simulink model "fullcontroller"  (R2024a)
settings: Solver=VariableStepAuto  StartTime=0.0  StopTime=5  RelTol=1e-3
undefined symbols (not defined in the file): al, al2, D, detect_delay, gear, J, K_b, K_t, Kp, kptr, kptr2, L, M, R, taud, taud2, taui, tautr, tautr2, Ts, wb, Wrad, wzi
settings Model: Creator=Emil  LastModifiedBy=Emil

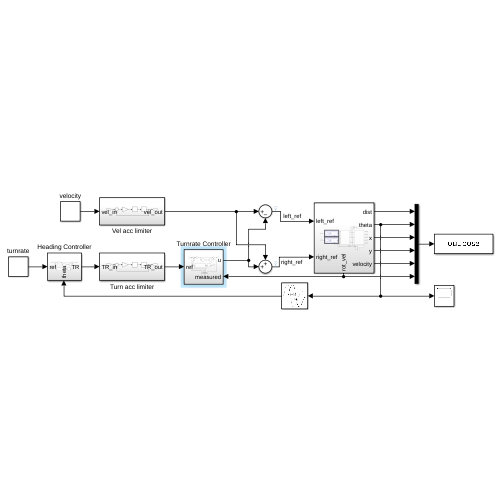
[thumbnail: Simulink's stored preview of the top-level diagram]
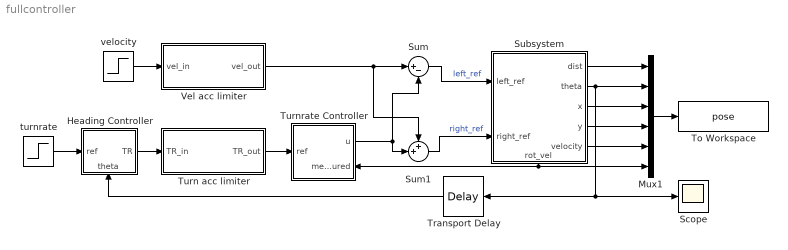
== system fullcontroller ==
  Heading Controller : Subsystem
      settings: PortSchema="{\"entries\":[{\"content\":{\"sides\":[{\"content\":{\"connectorIds\":[\"In1\"]},\"type\":\"ConnectorPlacement.EquallySpacedRectSide\",\"uuid\":\"b11ff20e-e335-4cf4-8322-1741fc0eb0d9\"},{\"content\":{\"connectorIds\":[\"Out1\"],\"side\":\"RIGHT\"},\"type\":\"ConnectorPlacement.EquallySpacedRectSide\",\"uuid\":\"fac384a7-55d1-4174-bfba-2626770ec520\"},{\"content\":{\"side\":\"TOP\"},\"type\":\"ConnectorPlacement.EquallySpacedRectSide\",\"uuid\":\"e325242d-1aa0-49ab-831d-5f009ebdd3a1\"},{\"content\":{\"connectorIds\":[\"In2\"],\"side\":\"BOTTOM\"},\"type\":\"ConnectorPlacement.EquallySpacedRectSide\",\"uuid\":\"ecba5a56-1e6f-49a1-b044-0798465cfff3\"}]},\"type\":\"ConnectorPlacement.EquallySpacedConnector\",\"uuid\":\"e06c607b-bc81-4732-8f37-206b6429b87f\"}],\"packageUris\":[\"http://schema.mathworks.com/mf0/Connector/R2020b\"],\"version\":\"1.0\"}"
  Mux1 : Mux  Inputs=6
  Scope : Scope
  Subsystem : Subsystem
      settings: PortSchema="{\"entries\":[{\"content\":{\"sides\":[{\"content\":{\"connectorIds\":[\"In1\",\"In2\"]},\"type\":\"ConnectorPlacement.EquallySpacedRectSide\",\"uuid\":\"e07b1068-606a-48e5-99f8-ac206fedc370\"},{\"content\":{\"connectorIds\":[\"Out1\",\"Out2\",\"Out3\",\"Out4\",\"Out5\"],\"side\":\"RIGHT\"},\"type\":\"ConnectorPlacement.EquallySpacedRectSide\",\"uuid\":\"74f7c964-e43c-4a5c-b857-64620296c31d\"},{\"content\":{\"side\":\"TOP\"},\"type\":\"ConnectorPlacement.EquallySpacedRectSide\",\"uuid\":\"331776cf-0fe9-40bc-a7d3-a5362462a3b4\"},{\"content\":{\"connectorIds\":[\"Out6\"],\"side\":\"BOTTOM\"},\"type\":\"ConnectorPlacement.EquallySpacedRectSide\",\"uuid\":\"defae528-7c87-433c-80d2-64239180a36e\"}]},\"type\":\"ConnectorPlacement.EquallySpacedConnector\",\"uuid\":\"4a46fe46-5a27-417e-b483-15ad12e25037\"}],\"packageUris\":[\"http://schema.mathworks.com/mf0/Connector/R2020b\"],\"version\":\"1.0\"}"
  Sum : Sum  Inputs=|+-
  Sum1 : Sum  Inputs=++|
  To Workspace : ToWorkspace  VariableName=pose  SaveFormat=Timeseries  SampleTime=-1
  Transport Delay : TransportDelay  DelayTime=detect_delay
  Turn acc limiter : Subsystem
  Turnrate Controller : Subsystem
      settings: PortSchema="{\"entries\":[{\"content\":{\"sides\":[{\"content\":{\"connectorIds\":[\"In1\"]},\"type\":\"ConnectorPlacement.EquallySpacedRectSide\",\"uuid\":\"51bc9059-e822-41b0-ad9a-58a8b0ba50e6\"},{\"content\":{\"connectorIds\":[\"Out1\",\"In2\"],\"side\":\"RIGHT\"},\"type\":\"ConnectorPlacement.EquallySpacedRectSide\",\"uuid\":\"f66c1df7-72f8-4460-aff3-9c1b28d487c9\"},{\"content\":{\"side\":\"TOP\"},\"type\":\"ConnectorPlacement.EquallySpacedRectSide\",\"uuid\":\"4a1b057f-a482-47d5-80e1-886b48e9d90a\"},{\"content\":{\"side\":\"BOTTOM\"},\"type\":\"ConnectorPlacement.EquallySpacedRectSide\",\"uuid\":\"a3ca5889-e809-4546-84f7-a1327d7aedb2\"}]},\"type\":\"ConnectorPlacement.EquallySpacedConnector\",\"uuid\":\"471e63b8-cc27-4ade-a003-f77fbe7d347a\"}],\"packageUris\":[\"http://schema.mathworks.com/mf0/Connector/R2020b\"],\"version\":\"1.0\"}"
  Vel acc limiter : Subsystem
  turnrate : Step  After=0.1  SampleTime=0
  velocity : Step  Time=0.05  After=0.1  SampleTime=0
  wires:
  Mux1/1 -> To Workspace/1
  Turn acc limiter/1(TR_out) -> Turnrate Controller/1(ref)
  velocity/1 -> Vel acc limiter/1(vel_in)
  Vel acc limiter/1(vel_out) -> Sum1/1, Sum/1
  Turnrate Controller/1(u) -> Sum1/2, Sum/2
  Sum/1 -> Subsystem/1(left_ref)  "left_ref"
  Sum1/1 -> Subsystem/2(right_ref)  "right_ref"
  Subsystem/1(dist) -> Mux1/1
  Subsystem/2(theta) -> Scope/1, Transport Delay/1, Mux1/2
  Subsystem/3(x) -> Mux1/3
  Subsystem/6(rot_vel) -> Turnrate Controller/2(measured), Mux1/6
  Subsystem/4(y) -> Mux1/4
  Subsystem/5(velocity) -> Mux1/5
  Heading Controller/1(TR) -> Turn acc limiter/1(TR_in)
  turnrate/1 -> Heading Controller/1(ref)
  Transport Delay/1 -> Heading Controller/2(theta)

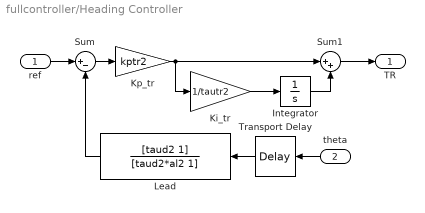
== system fullcontroller/Heading Controller ==
  ref : Inport
  theta : Inport  Port=2
  Integrator : Integrator
  Ki_tr : Gain  Gain=1/tautr2
  Kp_tr : Gain  Gain=kptr2
  Lead : TransferFcn  Numerator=[taud2 1]  Denominator=[taud2*al2 1]
  Sum : Sum  Inputs=|+-
  Sum1 : Sum  Inputs=|++
  Transport Delay : TransportDelay  DelayTime=detect_delay
  TR : Outport
  wires:
  theta/1 -> Transport Delay/1
  Transport Delay/1 -> Lead/1
  Lead/1 -> Sum/2
  Sum/1 -> Kp_tr/1
  Kp_tr/1 -> Sum1/1, Ki_tr/1
  Sum1/1 -> TR/1
  Ki_tr/1 -> Integrator/1
  Integrator/1 -> Sum1/2
  ref/1 -> Sum/1

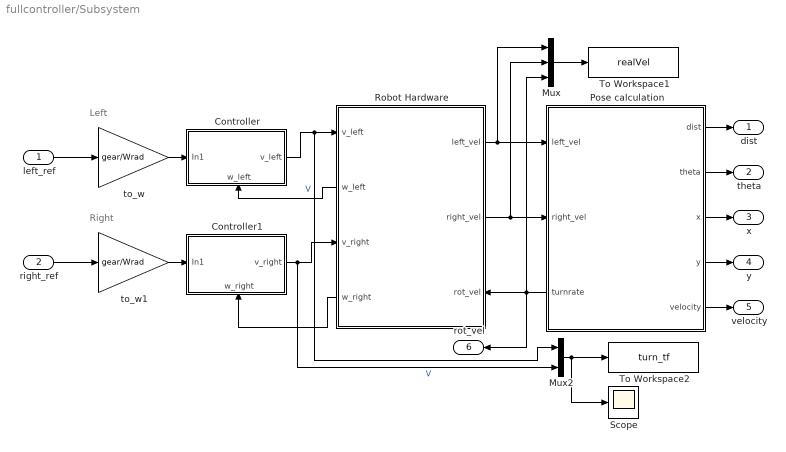
== system fullcontroller/Subsystem ==
  note: Left
  note: Right
  left_ref : Inport
  right_ref : Inport  Port=2
  Controller : Subsystem
      settings: PortSchema="{\"entries\":[{\"content\":{\"sides\":[{\"content\":{\"connectorIds\":[\"In1\"]},\"type\":\"ConnectorPlacement.EquallySpacedRectSide\",\"uuid\":\"2261268e-b6d1-4642-b5b2-9c0d266891c3\"},{\"content\":{\"connectorIds\":[\"Out1\"],\"side\":\"RIGHT\"},\"type\":\"ConnectorPlacement.EquallySpacedRectSide\",\"uuid\":\"4cfe3340-c893-4897-944b-2b0f290aa09a\"},{\"content\":{\"side\":\"TOP\"},\"type\":\"ConnectorPlacement.EquallySpacedRectSide\",\"uuid\":\"7108c253-9182-4668-b671-097ac861718f\"},{\"content\":{\"connectorIds\":[\"In2\"],\"side\":\"BOTTOM\"},\"type\":\"ConnectorPlacement.EquallySpacedRectSide\",\"uuid\":\"922d98a4-0301-4faa-ad82-d40d0b91da64\"}]},\"type\":\"ConnectorPlacement.EquallySpacedConnector\",\"uuid\":\"919d27b6-1b02-4194-927e-2efe9a2a427e\"}],\"packageUris\":[\"http://schema.mathworks.com/mf0/Connector/R2020b\"],\"version\":\"1.0\"}"
  Controller1 : Subsystem
      settings: PortSchema="{\"entries\":[{\"content\":{\"sides\":[{\"content\":{\"connectorIds\":[\"In1\"]},\"type\":\"ConnectorPlacement.EquallySpacedRectSide\",\"uuid\":\"2261268e-b6d1-4642-b5b2-9c0d266891c3\"},{\"content\":{\"connectorIds\":[\"Out1\"],\"side\":\"RIGHT\"},\"type\":\"ConnectorPlacement.EquallySpacedRectSide\",\"uuid\":\"4cfe3340-c893-4897-944b-2b0f290aa09a\"},{\"content\":{\"side\":\"TOP\"},\"type\":\"ConnectorPlacement.EquallySpacedRectSide\",\"uuid\":\"7108c253-9182-4668-b671-097ac861718f\"},{\"content\":{\"connectorIds\":[\"In2\"],\"side\":\"BOTTOM\"},\"type\":\"ConnectorPlacement.EquallySpacedRectSide\",\"uuid\":\"922d98a4-0301-4faa-ad82-d40d0b91da64\"}]},\"type\":\"ConnectorPlacement.EquallySpacedConnector\",\"uuid\":\"919d27b6-1b02-4194-927e-2efe9a2a427e\"}],\"packageUris\":[\"http://schema.mathworks.com/mf0/Connector/R2020b\"],\"version\":\"1.0\"}"
  Mux : Mux  Inputs=3
  Mux2 : Mux  Inputs=2
  Pose calculation : Subsystem
      settings: PortSchema="{\"entries\":[{\"content\":{\"sides\":[{\"content\":{\"connectorIds\":[\"In1\",\"In2\",\"Out6\"]},\"type\":\"ConnectorPlacement.EquallySpacedRectSide\",\"uuid\":\"bee664ca-7f8c-44aa-b52f-15284e139093\"},{\"content\":{\"connectorIds\":[\"Out1\",\"Out2\",\"Out3\",\"Out4\",\"Out5\"],\"side\":\"RIGHT\"},\"type\":\"ConnectorPlacement.EquallySpacedRectSide\",\"uuid\":\"08237290-c5a4-4af9-9089-e794091ff74a\"},{\"content\":{\"side\":\"TOP\"},\"type\":\"ConnectorPlacement.EquallySpacedRectSide\",\"uuid\":\"b1c152cf-47fe-475d-84d8-7839de8b0ea3\"}]},\"type\":\"ConnectorPlacement.EquallySpacedConnector\",\"uuid\":\"8442b5c9-5ac9-43e4-9044-7b6c0d0d80cf\"}],\"packageUris\":[\"http://schema.mathworks.com/mf0/Connector/R2020b\"],\"version\":\"1.0\"}"
  Robot Hardware : Subsystem
      settings: PortSchema="{\"entries\":[{\"content\":{\"sides\":[{\"content\":{\"connectorIds\":[\"In1\",\"Out3\",\"In2\",\"Out4\"]},\"type\":\"ConnectorPlacement.EquallySpacedRectSide\",\"uuid\":\"afaf08d4-5e01-48b3-8e5b-e3d507f44a91\"},{\"content\":{\"connectorIds\":[\"Out1\",\"Out2\",\"In3\"],\"side\":\"RIGHT\"},\"type\":\"ConnectorPlacement.EquallySpacedRectSide\",\"uuid\":\"2d9343fc-fd89-4bf8-9f3b-42343edd58e9\"},{\"content\":{\"side\":\"TOP\"},\"type\":\"ConnectorPlacement.EquallySpacedRectSide\",\"uuid\":\"dda2d7f6-2ea2-4182-90fb-cc6020acc35c\"}]},\"type\":\"ConnectorPlacement.EquallySpacedConnector\",\"uuid\":\"ab9e188f-2bc3-48d0-9cb1-1f465a1b570a\"}],\"packageUris\":[\"http://schema.mathworks.com/mf0/Connector/R2020b\"],\"version\":\"1.0\"}"
  Scope : Scope
  To Workspace1 : ToWorkspace  VariableName=realVel  SaveFormat=Timeseries  SampleTime=-1
  To Workspace2 : ToWorkspace  VariableName=turn_tf  SaveFormat=Timeseries  SampleTime=-1
  to_w : Gain  Gain=gear/Wrad
  to_w1 : Gain  Gain=gear/Wrad
  dist : Outport
  theta : Outport  Port=2
  x : Outport  Port=3
  y : Outport  Port=4
  velocity : Outport  Port=5
  rot_vel : Outport  Port=6
  wires:
  Pose calculation/3(x) -> x/1
  right_ref/1 -> to_w1/1
  Pose calculation/1(dist) -> dist/1
  Robot Hardware/2(right_vel) -> Mux/2, Pose calculation/2(right_vel)
  Robot Hardware/3(w_left) -> Controller/2(w_left)
  Pose calculation/2(theta) -> theta/1
  Controller/1(v_left) -> Mux2/1, Robot Hardware/1(v_left)  "V"
  Pose calculation/6(turnrate) -> rot_vel/1, Robot Hardware/3(rot_vel), Mux/3
  Pose calculation/4(y) -> y/1
  left_ref/1 -> to_w/1
  Mux2/1 -> Scope/1, To Workspace2/1
  to_w1/1 -> Controller1/1(In1)
  Robot Hardware/4(w_right) -> Controller1/2(w_right)
  Mux/1 -> To Workspace1/1
  to_w/1 -> Controller/1(In1)
  Controller1/1(v_right) -> Mux2/2, Robot Hardware/2(v_right)  "V"
  Robot Hardware/1(left_vel) -> Mux/1, Pose calculation/1(left_vel)
  Pose calculation/5(velocity) -> velocity/1

== system fullcontroller/Turn acc limiter ==
  TR_in : Inport
  Gain : Gain  Gain=100
  Integrator : Integrator
  Saturation : Saturate  UpperLimit=15  LowerLimit=-15
  Sum : Sum  Inputs=|+-
  TR_out : Outport
  wires:
  Sum/1 -> Gain/1
  Gain/1 -> Saturation/1
  Saturation/1 -> Integrator/1
  Integrator/1 -> Sum/2, TR_out/1
  TR_in/1 -> Sum/1

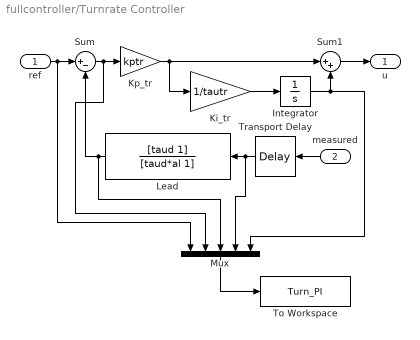
== system fullcontroller/Turnrate Controller ==
  ref : Inport
  measured : Inport  Port=2
  Integrator : Integrator
  Ki_tr : Gain  Gain=1/tautr
  Kp_tr : Gain  Gain=kptr
  Lead : TransferFcn  Numerator=[taud 1]  Denominator=[taud*al 1]
  Mux : Mux  Inputs=5
  Sum : Sum  Inputs=|+-
  Sum1 : Sum  Inputs=|++
  To Workspace : ToWorkspace  VariableName=Turn_PI  SaveFormat=Timeseries  SampleTime=-1
  Transport Delay : TransportDelay  DelayTime=detect_delay
  u : Outport
  wires:
  ref/1 -> Mux/1, Sum/1
  measured/1 -> Transport Delay/1
  Transport Delay/1 -> Mux/4, Lead/1
  Lead/1 -> Mux/3, Sum/2
  Sum/1 -> Mux/2, Kp_tr/1
  Ki_tr/1 -> Integrator/1
  Integrator/1 -> Mux/5, Sum1/2
  Kp_tr/1 -> Ki_tr/1, Sum1/1
  Sum1/1 -> u/1
  Mux/1 -> To Workspace/1

== system fullcontroller/Vel acc limiter ==
  vel_in : Inport
  Gain : Gain  Gain=100
  Integrator : Integrator
  Saturation : Saturate  UpperLimit=3  LowerLimit=-3
  Sum : Sum  Inputs=|+-
  vel_out : Outport
  wires:
  Sum/1 -> Gain/1
  Gain/1 -> Saturation/1
  Saturation/1 -> Integrator/1
  Integrator/1 -> Sum/2, vel_out/1
  vel_in/1 -> Sum/1

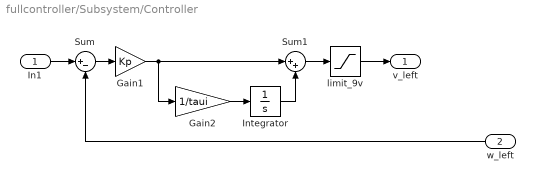
== system fullcontroller/Subsystem/Controller ==
  In1 : Inport
  w_left : Inport  Port=2
  Gain1 : Gain  Gain=Kp
  Gain2 : Gain  Gain=1/taui
  Integrator : Integrator
  Sum : Sum  Inputs=|+-
  Sum1 : Sum  Inputs=|++
  limit_9v : Saturate  UpperLimit=9  LowerLimit=-9
  v_left : Outport
  wires:
  Gain1/1 -> Gain2/1, Sum1/1
  Gain2/1 -> Integrator/1
  Sum1/1 -> limit_9v/1
  Sum/1 -> Gain1/1
  In1/1 -> Sum/1
  w_left/1 -> Sum/2
  Integrator/1 -> Sum1/2
  limit_9v/1 -> v_left/1

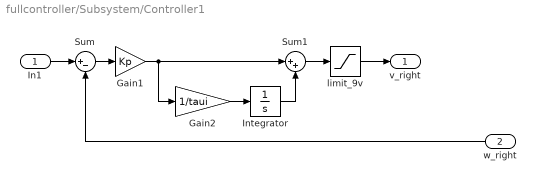
== system fullcontroller/Subsystem/Controller1 ==
  In1 : Inport
  w_right : Inport  Port=2
  Gain1 : Gain  Gain=Kp
  Gain2 : Gain  Gain=1/taui
  Integrator : Integrator
  Sum : Sum  Inputs=|+-
  Sum1 : Sum  Inputs=|++
  limit_9v : Saturate  UpperLimit=9  LowerLimit=-9
  v_right : Outport
  wires:
  Gain1/1 -> Gain2/1, Sum1/1
  Gain2/1 -> Integrator/1
  Sum1/1 -> limit_9v/1
  Sum/1 -> Gain1/1
  In1/1 -> Sum/1
  w_right/1 -> Sum/2
  Integrator/1 -> Sum1/2
  limit_9v/1 -> v_right/1

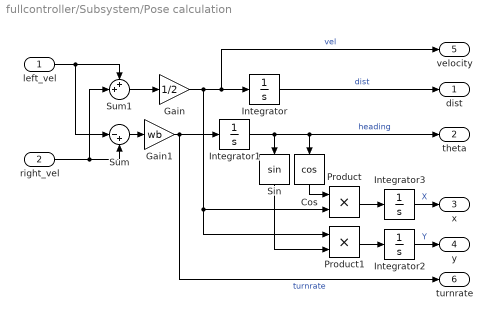
== system fullcontroller/Subsystem/Pose calculation ==
  left_vel : Inport
  right_vel : Inport  Port=2
  Cos : Trigonometry  Operator=cos
  Gain : Gain  Gain=1/2
  Gain1 : Gain  Gain=wb
  Integrator{,1..3} (4 alike) : Integrator
  Product : Product
  Product1 : Product
  Sin : Trigonometry
  Sum : Sum  Inputs=|-+
  Sum1 : Sum  Inputs=++|
  dist : Outport
  theta : Outport  Port=2
  x : Outport  Port=3
  y : Outport  Port=4
  velocity : Outport  Port=5
  turnrate : Outport  Port=6
  wires:
  Gain/1 -> Product/2, Product1/1, velocity/1, Integrator/1  "vel"
  Integrator/1 -> dist/1  "dist"
  left_vel/1 -> Sum1/1, Sum/1
  right_vel/1 -> Sum/2, Sum1/2
  Sum1/1 -> Gain/1
  Sum/1 -> Gain1/1
  Gain1/1 -> Integrator1/1, turnrate/1  "turnrate"
  Integrator1/1 -> Sin/1, Cos/1, theta/1  "heading"
  Product1/1 -> Integrator2/1
  Product/1 -> Integrator3/1
  Cos/1 -> Product/1
  Sin/1 -> Product1/2
  Integrator3/1 -> x/1  "X"
  Integrator2/1 -> y/1  "Y"

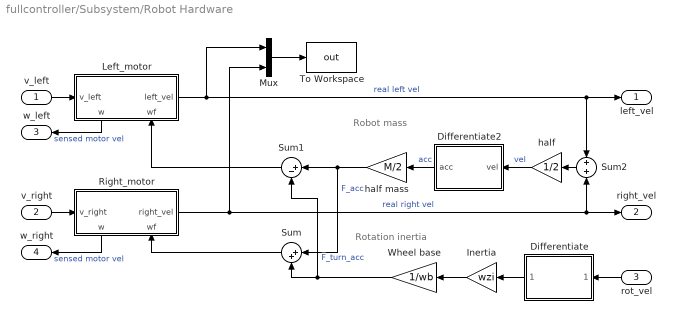
== system fullcontroller/Subsystem/Robot Hardware ==
  note: Robot mass
  note: Rotation inertia
  v_left : Inport
  v_right : Inport  Port=2
  rot_vel : Inport  Port=3
  Differentiate : Subsystem
  Differentiate2 : Subsystem
  Inertia : Gain  Gain=wzi
  Left_motor : Subsystem
      settings: PortSchema="{\"entries\":[{\"content\":{\"sides\":[{\"content\":{\"connectorIds\":[\"In1\"]},\"type\":\"ConnectorPlacement.EquallySpacedRectSide\",\"uuid\":\"70979ced-7f5f-49af-9b2c-3d9d1d67e998\"},{\"content\":{\"connectorIds\":[\"Out1\"],\"side\":\"RIGHT\"},\"type\":\"ConnectorPlacement.EquallySpacedRectSide\",\"uuid\":\"da077ec4-3f52-42e4-91c7-0922f19146a5\"},{\"content\":{\"side\":\"TOP\"},\"type\":\"ConnectorPlacement.EquallySpacedRectSide\",\"uuid\":\"05153d0d-0b42-4382-a094-d2758cc8283e\"},{\"content\":{\"connectorIds\":[\"Out2\",\"In2\"],\"side\":\"BOTTOM\"},\"type\":\"ConnectorPlacement.EquallySpacedRectSide\",\"uuid\":\"5b7bf5e4-9b0e-482f-a660-11d73d69e90a\"}]},\"type\":\"ConnectorPlacement.EquallySpacedConnector\",\"uuid\":\"fd374a38-0724-4b07-a862-27e38a23ae30\"}],\"packageUris\":[\"http://schema.mathworks.com/mf0/Connector/R2020b\"],\"version\":\"1.0\"}"
  Mux : Mux  Inputs=2
  Right_motor : Subsystem
      settings: PortSchema="{\"entries\":[{\"content\":{\"sides\":[{\"content\":{\"connectorIds\":[\"In1\"]},\"type\":\"ConnectorPlacement.EquallySpacedRectSide\",\"uuid\":\"70979ced-7f5f-49af-9b2c-3d9d1d67e998\"},{\"content\":{\"connectorIds\":[\"Out1\"],\"side\":\"RIGHT\"},\"type\":\"ConnectorPlacement.EquallySpacedRectSide\",\"uuid\":\"da077ec4-3f52-42e4-91c7-0922f19146a5\"},{\"content\":{\"side\":\"TOP\"},\"type\":\"ConnectorPlacement.EquallySpacedRectSide\",\"uuid\":\"05153d0d-0b42-4382-a094-d2758cc8283e\"},{\"content\":{\"connectorIds\":[\"Out2\",\"In2\"],\"side\":\"BOTTOM\"},\"type\":\"ConnectorPlacement.EquallySpacedRectSide\",\"uuid\":\"5b7bf5e4-9b0e-482f-a660-11d73d69e90a\"}]},\"type\":\"ConnectorPlacement.EquallySpacedConnector\",\"uuid\":\"fd374a38-0724-4b07-a862-27e38a23ae30\"}],\"packageUris\":[\"http://schema.mathworks.com/mf0/Connector/R2020b\"],\"version\":\"1.0\"}"
  Sum : Sum  Inputs=|++
  Sum1 : Sum  Inputs=|+-
  Sum2 : Sum  Inputs=+|+
  To Workspace : ToWorkspace  VariableName=out  SaveFormat=Timeseries  SampleTime=-1
  Wheel base : Gain  Gain=1/wb
  half : Gain  Gain=1/2
  half mass : Gain  Gain=M/2
  left_vel : Outport
  right_vel : Outport  Port=2
  w_left : Outport  Port=3
  w_right : Outport  Port=4
  wires:
  v_left/1 -> Left_motor/1(v_left)
  Left_motor/1(left_vel) -> Mux/1, Sum2/1, left_vel/1  "real left vel"
  Left_motor/2(w) -> w_left/1  "sensed motor vel"
  v_right/1 -> Right_motor/1(v_right)
  Right_motor/2(w) -> w_right/1  "sensed motor vel"
  Right_motor/1(right_vel) -> Mux/2, Sum2/2, right_vel/1  "real right vel"
  Differentiate/1(rot_acc) -> Inertia/1
  Inertia/1 -> Wheel base/1
  rot_vel/1 -> Differentiate/1(rot_vel)
  Mux/1 -> To Workspace/1
  half/1 -> Differentiate2/1(vel)  "vel"
  Sum2/1 -> half/1
  Differentiate2/1(acc) -> half mass/1  "acc"
  half mass/1 -> Sum/1, Sum1/1  "F_acc"
  Wheel base/1 -> Sum/2, Sum1/2  "F_turn_acc"
  Sum/1 -> Right_motor/2(wf)
  Sum1/1 -> Left_motor/2(wf)

== system fullcontroller/Subsystem/Robot Hardware/Differentiate ==
  rot_vel : Inport
  Gain : Gain  Gain=100
  Integrator : Integrator
  Sum : Sum  Inputs=|+-
  heading_acc : Scope
  rot_acc : Outport
  wires:
  rot_vel/1 -> Sum/1
  Sum/1 -> Gain/1  "e"
  Integrator/1 -> Sum/2
  Gain/1 -> heading_acc/1, Integrator/1, rot_acc/1

== system fullcontroller/Subsystem/Robot Hardware/Differentiate2 ==
  vel : Inport
  Gain : Gain  Gain=100
  Integrator : Integrator
  Sum : Sum  Inputs=|+-
  heading_acc : Scope
  acc : Outport
  wires:
  vel/1 -> Sum/1
  Sum/1 -> Gain/1  "e"
  Integrator/1 -> Sum/2
  Gain/1 -> heading_acc/1, Integrator/1, acc/1

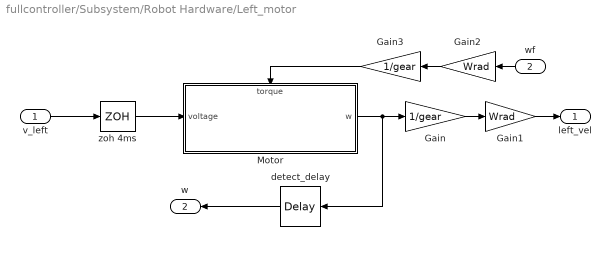
== system fullcontroller/Subsystem/Robot Hardware/Left_motor ==
  v_left : Inport
  wf : Inport  Port=2
  Gain : Gain  Gain=1/gear
  Gain1 : Gain  Gain=Wrad
  Gain2 : Gain  Gain=Wrad
  Gain3 : Gain  Gain=1/gear
  Motor : Subsystem
      settings: PortSchema="{\"entries\":[{\"content\":{\"sides\":[{\"content\":{\"connectorIds\":[\"In1\"]},\"type\":\"ConnectorPlacement.EquallySpacedRectSide\",\"uuid\":\"70979ced-7f5f-49af-9b2c-3d9d1d67e998\"},{\"content\":{\"connectorIds\":[\"Out1\"],\"side\":\"RIGHT\"},\"type\":\"ConnectorPlacement.EquallySpacedRectSide\",\"uuid\":\"da077ec4-3f52-42e4-91c7-0922f19146a5\"},{\"content\":{\"connectorIds\":[\"In2\"],\"side\":\"TOP\"},\"type\":\"ConnectorPlacement.EquallySpacedRectSide\",\"uuid\":\"05153d0d-0b42-4382-a094-d2758cc8283e\"}]},\"type\":\"ConnectorPlacement.EquallySpacedConnector\",\"uuid\":\"fd374a38-0724-4b07-a862-27e38a23ae30\"}],\"packageUris\":[\"http://schema.mathworks.com/mf0/Connector/R2020b\"],\"version\":\"1.0\"}"
  detect_delay : TransportDelay  DelayTime=detect_delay
  zoh 4ms : ZeroOrderHold  SampleTime=Ts
  left_vel : Outport
  w : Outport  Port=2
  wires:
  Gain/1 -> Gain1/1
  Gain2/1 -> Gain3/1
  Gain1/1 -> left_vel/1
  wf/1 -> Gain2/1
  Gain3/1 -> Motor/2(torque)
  v_left/1 -> zoh 4ms/1
  zoh 4ms/1 -> Motor/1(voltage)
  detect_delay/1 -> w/1
  Motor/1(w) -> detect_delay/1, Gain/1

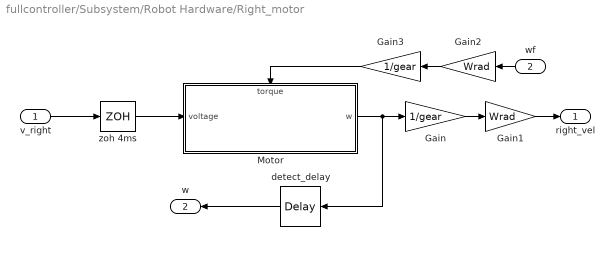
== system fullcontroller/Subsystem/Robot Hardware/Right_motor ==
  v_right : Inport
  wf : Inport  Port=2
  Gain : Gain  Gain=1/gear
  Gain1 : Gain  Gain=Wrad
  Gain2 : Gain  Gain=Wrad
  Gain3 : Gain  Gain=1/gear
  Motor : Subsystem
      settings: PortSchema="{\"entries\":[{\"content\":{\"sides\":[{\"content\":{\"connectorIds\":[\"In1\"]},\"type\":\"ConnectorPlacement.EquallySpacedRectSide\",\"uuid\":\"70979ced-7f5f-49af-9b2c-3d9d1d67e998\"},{\"content\":{\"connectorIds\":[\"Out1\"],\"side\":\"RIGHT\"},\"type\":\"ConnectorPlacement.EquallySpacedRectSide\",\"uuid\":\"da077ec4-3f52-42e4-91c7-0922f19146a5\"},{\"content\":{\"connectorIds\":[\"In2\"],\"side\":\"TOP\"},\"type\":\"ConnectorPlacement.EquallySpacedRectSide\",\"uuid\":\"05153d0d-0b42-4382-a094-d2758cc8283e\"}]},\"type\":\"ConnectorPlacement.EquallySpacedConnector\",\"uuid\":\"fd374a38-0724-4b07-a862-27e38a23ae30\"}],\"packageUris\":[\"http://schema.mathworks.com/mf0/Connector/R2020b\"],\"version\":\"1.0\"}"
  detect_delay : TransportDelay  DelayTime=detect_delay
  zoh 4ms : ZeroOrderHold  SampleTime=Ts
  right_vel : Outport
  w : Outport  Port=2
  wires:
  Gain/1 -> Gain1/1
  Gain2/1 -> Gain3/1
  Gain1/1 -> right_vel/1
  wf/1 -> Gain2/1
  Gain3/1 -> Motor/2(torque)
  v_right/1 -> zoh 4ms/1
  zoh 4ms/1 -> Motor/1(voltage)
  detect_delay/1 -> w/1
  Motor/1(w) -> detect_delay/1, Gain/1

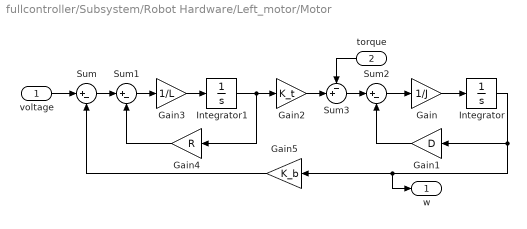
== system fullcontroller/Subsystem/Robot Hardware/Left_motor/Motor ==
  voltage : Inport
  torque : Inport  Port=2
  Gain : Gain  Gain=1/J
  Gain1 : Gain  Gain=D
  Gain2 : Gain  Gain=K_t
  Gain3 : Gain  Gain=1/L
  Gain4 : Gain  Gain=R
  Gain5 : Gain  Gain=K_b
  Integrator : Integrator
  Integrator1 : Integrator
  Sum : Sum  Inputs=|+-
  Sum1 : Sum  Inputs=|+-
  Sum2 : Sum  Inputs=|+-
  Sum3 : Sum  Inputs=-+|
  w : Outport
  wires:
  voltage/1 -> Sum/1
  Sum/1 -> Sum1/1
  torque/1 -> Sum3/1
  Sum3/1 -> Sum2/1
  Sum2/1 -> Gain/1
  Gain3/1 -> Integrator1/1
  Integrator1/1 -> Gain4/1, Gain2/1
  Gain2/1 -> Sum3/2
  Sum1/1 -> Gain3/1
  Gain4/1 -> Sum1/2
  Gain/1 -> Integrator/1
  Integrator/1 -> w/1, Gain5/1, Gain1/1
  Gain1/1 -> Sum2/2
  Gain5/1 -> Sum/2

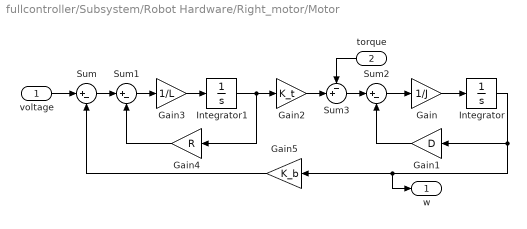
== system fullcontroller/Subsystem/Robot Hardware/Right_motor/Motor ==
  voltage : Inport
  torque : Inport  Port=2
  Gain : Gain  Gain=1/J
  Gain1 : Gain  Gain=D
  Gain2 : Gain  Gain=K_t
  Gain3 : Gain  Gain=1/L
  Gain4 : Gain  Gain=R
  Gain5 : Gain  Gain=K_b
  Integrator : Integrator
  Integrator1 : Integrator
  Sum : Sum  Inputs=|+-
  Sum1 : Sum  Inputs=|+-
  Sum2 : Sum  Inputs=|+-
  Sum3 : Sum  Inputs=-+|
  w : Outport
  wires:
  voltage/1 -> Sum/1
  Sum/1 -> Sum1/1
  torque/1 -> Sum3/1
  Sum3/1 -> Sum2/1
  Sum2/1 -> Gain/1
  Gain3/1 -> Integrator1/1
  Integrator1/1 -> Gain4/1, Gain2/1
  Gain2/1 -> Sum3/2
  Sum1/1 -> Gain3/1
  Gain4/1 -> Sum1/2
  Gain/1 -> Integrator/1
  Integrator/1 -> w/1, Gain5/1, Gain1/1
  Gain1/1 -> Sum2/2
  Gain5/1 -> Sum/2
